simulink model "sample_step4"  (R2021b)
settings: Solver=VariableStepAuto  StartTime=0.0  StopTime=5  RelTol=1e-3
settings Model: Creator=kawata  LastModifiedBy=kawata

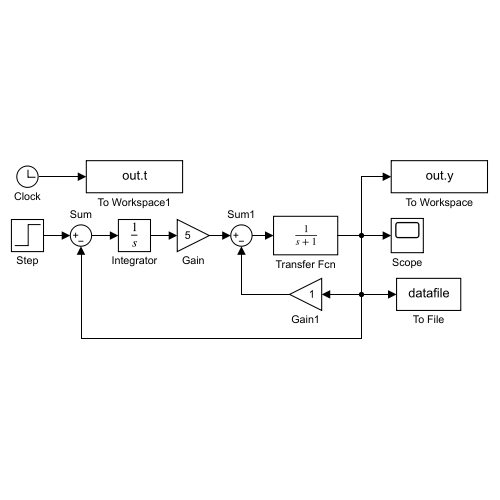
[thumbnail: Simulink's stored preview of the top-level diagram]
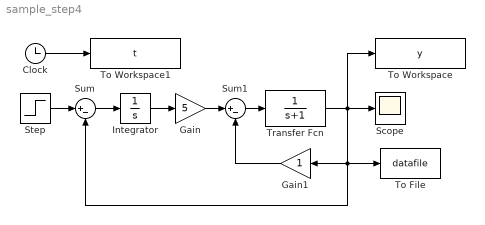
== system sample_step4 ==
  Clock : Clock
  Gain : Gain  Gain=5
  Gain1 : Gain
  Integrator : Integrator
  Scope : Scope
  Step : Step  SampleTime=0
  Sum : Sum  Inputs=|+-
  Sum1 : Sum  Inputs=|+-
  To File : ToFile  Filename=datafile  MatrixName=output  SaveFormat=Timeseries
  To Workspace : ToWorkspace  VariableName=y  SampleTime=-1
  To Workspace1 : ToWorkspace  VariableName=t  SampleTime=-1
  Transfer Fcn : TransferFcn  Denominator=[1 1]
  wires:
  Clock/1 -> To Workspace1/1
  Gain1/1 -> Sum1/2
  Integrator/1 -> Gain/1
  Transfer Fcn/1 -> To Workspace/1, Scope/1, To File/1, Gain1/1, Sum/2
  Sum/1 -> Integrator/1
  Step/1 -> Sum/1
  Gain/1 -> Sum1/1
  Sum1/1 -> Transfer Fcn/1
